simulink model "mavsim_chap5"  (R2017a)
settings: Solver=ode45  StartTime=0.0  StopTime=150  RelTol=1e-3  EnableMultiTasking=on
InitFcn:
  | param_chap5
undefined symbols (not defined in the file or in its folder): drawAircraft_chap5, P, plotmavstatevariables, traj_helix, traj_line
libraries: aerolibanimutils x1
settings Model: Creator=beard  LastModifiedBy=STAN
settings DataIOCC: LimitDataPoints=on  SaveFormat=Array  SignalLoggingSaveFormat=ModelDataLogs
settings OptimizationCC: ExpressionDepthLimit=2147483647  InitFltsAndDblsToZero=on  LifeSpan=inf
settings DebuggingCC: UnderspecifiedInitializationDetection=Classic  MergeDetectMultiDrivingBlocksExec=none  SolverPrmCheckMsg=warning  FcnCallInpInsideContextMsg=warning  StateNameClashWarn=warning  SFUnexpectedBacktrackingDiag=warning  SFNoUnconditionalDefaultTransitionDiag=warning  SFExecutionAtInitializationDiag=none
settings HardwareCC: ProdBitPerPointer=32  ProdBitPerSizeT=32  ProdBitPerPtrDiffT=32  ProdLargestAtomicFloat=None  ProdIntDivRoundTo=Undefined  ProdEndianess=Unspecified  ProdWordSize=32  ProdHWDeviceType=32-bit Generic
settings ModelReferenceCC: PropagateSignalLabelsOutOfModel=off
settings GRTTargetCC: TargetLangStandard=C89/C90 (ANSI)  GeneratePreprocessorConditionals=Disable all  CombineOutputUpdateFcns=off  GRTInterface=on
settings ConfigComp: CovMetricSettings=dw  CovHtmlReporting=on  CovSaveCumulativeToWorkspaceVar=on  CovSaveSingleToWorkspaceVar=on  CovExternalEMLEnable=off  CovSFcnEnable=off

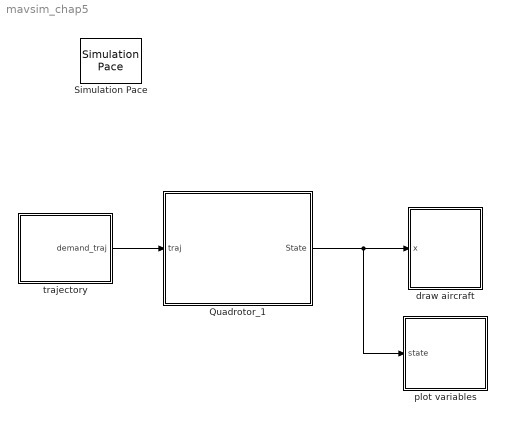
== system mavsim_chap5 ==
  Quadrotor_1 : Subsystem
      mask Display: image('Qcopter.jpg');
  Simulation Pace : aerolibanimutils/Simulation Pace  SimulationPace=1  SleepMode=MATLAB Thread  OutputPaceError=off  SampleTime=1/100
  draw aircraft : Subsystem
      mask Display: image(imread('tv.jpg'))
  plot variables : Subsystem
  trajectory : Subsystem
  wires:
  trajectory/1(demand_traj) -> Quadrotor_1/1(traj)
  Quadrotor_1/1(State) -> plot variables/1(state), draw aircraft/1(x)

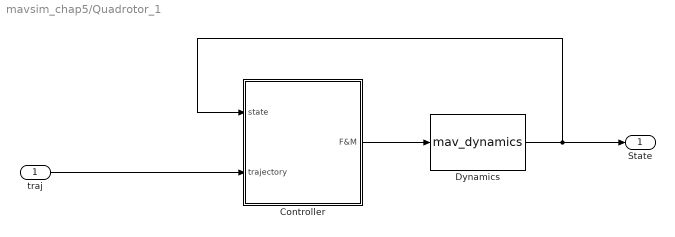
== system mavsim_chap5/Quadrotor_1 ==
  traj : Inport
  Controller : Subsystem
  Dynamics : S-Function  FunctionName=mav_dynamics  Parameters=P  SFunctionDeploymentMode=off  EnableBusSupport=off
  State : Outport
  wires:
  Dynamics/1 -> Controller/1(state), State/1
  traj/1 -> Controller/2(trajectory)
  Controller/1(F&M) -> Dynamics/1

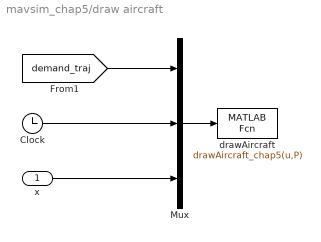
== system mavsim_chap5/draw aircraft ==
  x : Inport
  Clock : Clock
  Mux : Mux  Inputs=3
  drawAircraft : MATLABFcn  MATLABFcn=drawAircraft_chap5(u,P)  OutputDimensions=0  SampleTime=0.1
  wires:
  Mux/1 -> drawAircraft/1
  x/1 -> Mux/3
  Clock/1 -> Mux/2
  [demand_traj] -> Mux/1

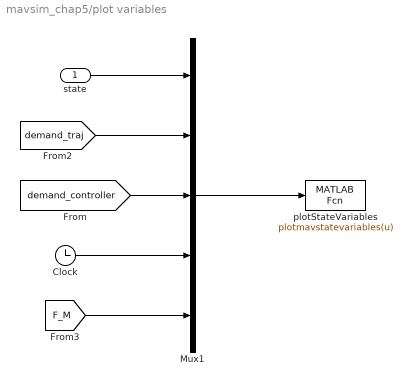
== system mavsim_chap5/plot variables ==
  state : Inport
  Clock : Clock
  Mux1 : Mux  Inputs=5
  plotStateVariables : MATLABFcn  MATLABFcn=plotmavstatevariables(u)  OutputDimensions=0  SampleTime=0.1
  wires:
  state/1 -> Mux1/1
  Clock/1 -> Mux1/4
  [demand_controller] -> Mux1/3
  [F_M] -> Mux1/5
  [demand_traj] -> Mux1/2
  Mux1/1 -> plotStateVariables/1

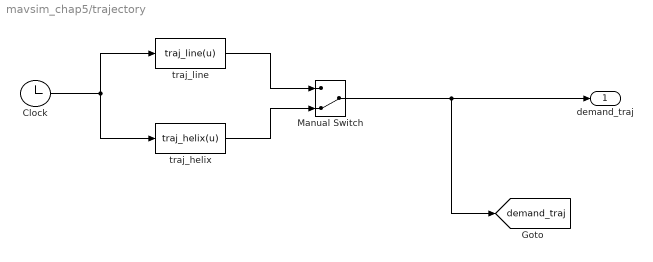
== system mavsim_chap5/trajectory ==
  Clock : Clock
  Manual Switch : ManualSwitch  CurrentSetting=0
  traj_helix : MATLABFcn  MATLABFcn=traj_helix(u)  OutputDimensions=11
  traj_line : MATLABFcn  MATLABFcn=traj_line(u)  OutputDimensions=11
  demand_traj : Outport
  tag scope: demand_traj=global
  wires:
  Manual Switch/1 -> demand_traj/1, [demand_traj]
  Clock/1 -> traj_helix/1, traj_line/1
  traj_line/1 -> Manual Switch/1
  traj_helix/1 -> Manual Switch/2

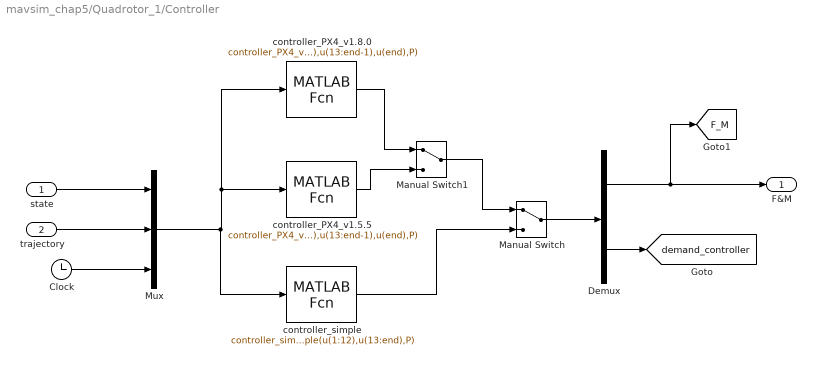
== system mavsim_chap5/Quadrotor_1/Controller ==
  state : Inport
  trajectory : Inport  Port=2
  Clock : Clock
  Demux : Demux  Outputs=[4;9]
  Manual Switch : ManualSwitch
  Manual Switch1 : ManualSwitch
  Mux : Mux  Inputs=3
  controller_PX4_v1.5.5 : MATLABFcn  MATLABFcn=controller_PX4_v1_5_5(u(1:12),u(13:end-1),u(end),P)  OutputDimensions=13
  controller_PX4_v1.8.0 : MATLABFcn  MATLABFcn=controller_PX4_v1_8_0(u(1:12),u(13:end-1),u(end),P)  OutputDimensions=13
  controller_simple : MATLABFcn  MATLABFcn=controller_simple(u(1:12),u(13:end),P)
  F&M : Outport
  tag scope: F_M=global, demand_controller=global
  wires:
  controller_PX4_v1.8.0/1 -> Manual Switch1/1
  trajectory/1 -> Mux/2
  state/1 -> Mux/1
  Manual Switch/1 -> Demux/1
  controller_simple/1 -> Manual Switch/2
  Demux/1 -> [F_M], F&M/1
  Demux/2 -> [demand_controller]
  Clock/1 -> Mux/3
  controller_PX4_v1.5.5/1 -> Manual Switch1/2
  Manual Switch1/1 -> Manual Switch/1
  Mux/1 -> controller_PX4_v1.8.0/1, controller_PX4_v1.5.5/1, controller_simple/1
